simulink model "RotationalPendulum_Nonlinear"  (R2025b)
settings: Solver=VariableStepAuto  StartTime=0.0  StopTime=10  RelTol=1e-3
values from neighbouring files (symbols this model uses):
  eps_v1 = 0.02    [build_sysid_parameters.m]
  eps_v2 = 0.02    [build_sysid_parameters.m]
  p_0 = 0    [build_sysid_parameters.m]
  p_alpha = 33.6175    [build_sysid_parameters.m]
  p_b1 = 744.5341    [build_sysid_parameters.m]
  p_b2 = 0.0670    (= 0.067)    [build_sysid_parameters.m]
  p_c = (l_1 / g) * p_g2    (= 1.14196432212)    [build_sysid_parameters.m]
  p_c1 = 23.9089    [build_sysid_parameters.m]
  p_c2 = 0.2491    [build_sysid_parameters.m]
  p_g1 = 105.6867    [build_sysid_parameters.m]
  p_g2 = 112.0267    [build_sysid_parameters.m]
  p_s_d2 = 0.1836    [build_sysid_parameters.m]
  p_u = 4091.4423    [build_sysid_parameters.m]
  v_s2 = 3.5000    (= 3.5)    [build_sysid_parameters.m]
undefined symbols (not defined in the file or in its folder): theta_1_0_mask, theta_1_dot_0_mask, theta_2_0_mask, theta_2_dot_0_mask
settings Model: Creator=djangovanderplas  LastModifiedBy=thoma
settings DataIOCC: ExternalInput=inputData

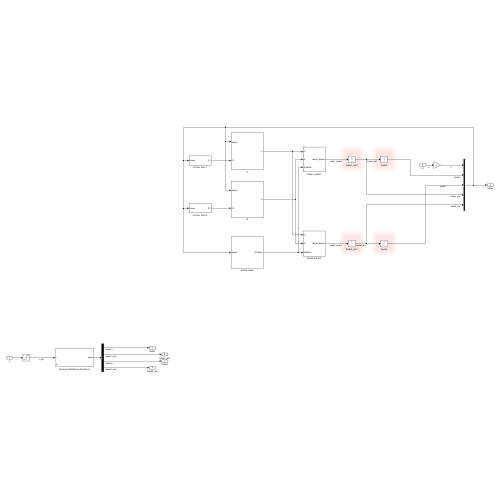
[thumbnail: Simulink's stored preview of the top-level diagram]
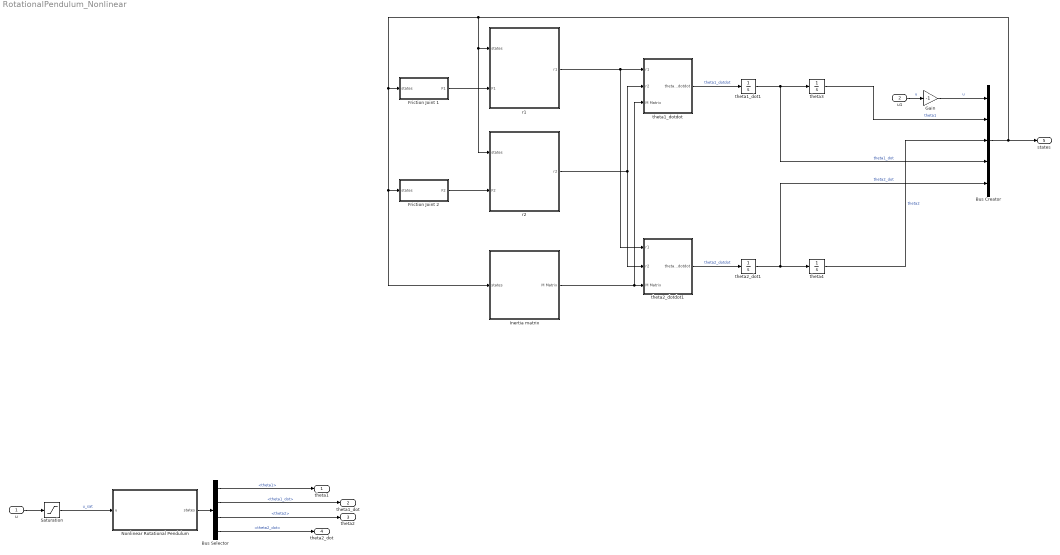
== system RotationalPendulum_Nonlinear ==
  u : Inport
  u1 : Inport  Port=2
  Bus Creator : BusCreator  Inputs=5
  Bus Selector : BusSelector  OutputSignals=theta1,theta1_dot,theta2,theta2_dot
  Friction Joint 1 : Subsystem
  Friction Joint 2 : Subsystem
  Gain : Gain  Gain=-1
  Inertia matrix : Subsystem
  Nonlinear Rotational Pendulum : Subsystem  mask{theta_1_0_mask=pi+0.1, theta_2_0_mask=0, theta_1_dot_0_mask=0, theta_2_dot_0_mask=0}
      mask prompts: theta_1_0_mask "Initial \theta_1 [rad]"; theta_2_0_mask "Initial \theta_2 [rad]"; theta_1_dot_0_mask "Initial \dot\theta_1 [rad]"; theta_2_dot_0_mask "Initial \dot\theta_1 [rad]"
  Saturation : Saturate  UpperLimit=1  LowerLimit=-1
  r1 : Subsystem
  r2 : Subsystem
  theta1_dot1 : Integrator  InitialCondition=theta_1_dot_0_mask
  theta1_dotdot : Subsystem
  theta2_dot1 : Integrator  InitialCondition=theta_2_dot_0_mask
  theta2_dotdot1 : Subsystem
  theta3 : Integrator  InitialCondition=theta_1_0_mask
  theta4 : Integrator  InitialCondition=theta_2_0_mask
  theta1 : Outport
  theta1_dot : Outport  Port=2
  theta2 : Outport  Port=3
  theta2_dot : Outport  Port=4
  states : Outport  Port=5
  wires:
  u/1 -> Saturation/1
  Nonlinear Rotational Pendulum/1(states) -> Bus Selector/1
  Bus Selector/1 -> theta1/1  "<theta1>"
  Bus Selector/3 -> theta2/1  "<theta2>"
  Bus Selector/2 -> theta1_dot/1  "<theta1_dot>"
  Bus Selector/4 -> theta2_dot/1  "<theta2_dot>"
  Saturation/1 -> Nonlinear Rotational Pendulum/1(u)  "u_sat"
  Inertia matrix/1(M Matrix) -> theta2_dotdot1/3(M Matrix), theta1_dotdot/3(M Matrix)
  u1/1 -> Gain/1  "u"
  Friction Joint 1/1(F1) -> r1/2(F1)
  Bus Creator/1 -> Friction Joint 2/1(states), Inertia matrix/1(states), Friction Joint 1/1(states), r1/1(states), r2/1(states), states/1
  theta3/1 -> Bus Creator/2  "theta1"
  theta2_dot1/1 -> theta4/1, Bus Creator/5  "theta2_dot"
  theta1_dotdot/1(theta1_dotdot) -> theta1_dot1/1  "theta1_dotdot"
  Gain/1 -> Bus Creator/1  "u"
  r1/1(r1) -> theta2_dotdot1/1(r1), theta1_dotdot/1(r1)
  theta4/1 -> Bus Creator/3  "theta2"
  r2/1(r2) -> theta2_dotdot1/2(r2), theta1_dotdot/2(r2)
  theta1_dot1/1 -> Bus Creator/4, theta3/1  "theta1_dot"
  Friction Joint 2/1(F2) -> r2/2(F2)
  theta2_dotdot1/1(theta2_dotdot) -> theta2_dot1/1  "theta2_dotdot"

== system RotationalPendulum_Nonlinear/Friction Joint 1 ==
  states : Inport
  Add : Sum
  Bus Selector : BusSelector  OutputSignals=theta1_dot
  Gain : Gain  Gain=p_b1
  Gain1 : Gain  Gain=1/eps_v1
  Gain2 : Gain  Gain=p_c1
  Tanh : Trigonometry  Operator=tanh
  F1 : Outport
  wires:
  states/1 -> Bus Selector/1
  Gain1/1 -> Tanh/1
  Tanh/1 -> Gain2/1
  Add/1 -> F1/1
  Gain2/1 -> Add/1
  Gain/1 -> Add/2
  Bus Selector/1 -> Gain1/1, Gain/1  "<theta1_dot>"

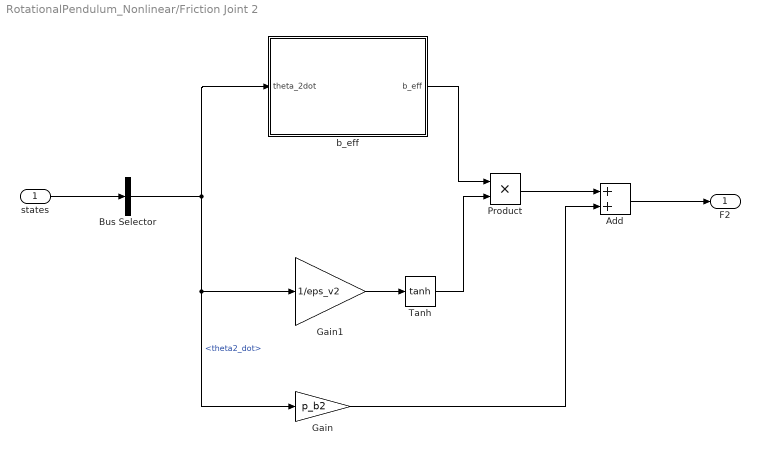
== system RotationalPendulum_Nonlinear/Friction Joint 2 ==
  states : Inport
  Add : Sum
  Bus Selector : BusSelector  OutputSignals=theta2_dot
  Gain : Gain  Gain=p_b2
  Gain1 : Gain  Gain=1/eps_v2
  Product : Product
  Tanh : Trigonometry  Operator=tanh
  b_eff : Subsystem
  F2 : Outport
  wires:
  Bus Selector/1 -> b_eff/1(theta_2dot), Gain/1, Gain1/1  "<theta2_dot>"
  Gain1/1 -> Tanh/1
  Tanh/1 -> Product/2
  Add/1 -> F2/1
  states/1 -> Bus Selector/1
  b_eff/1(b_eff) -> Product/1
  Product/1 -> Add/1
  Gain/1 -> Add/2

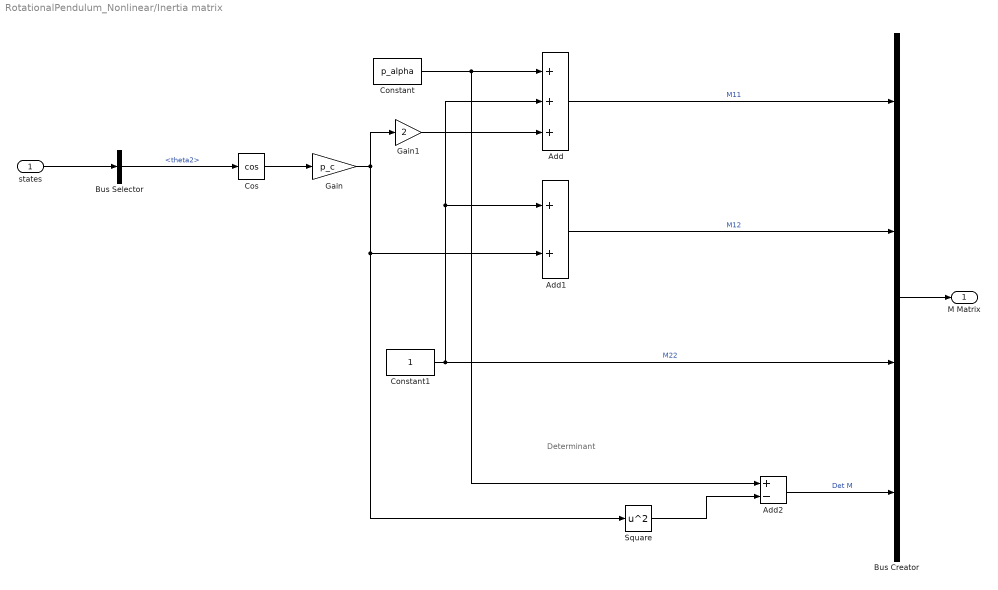
== system RotationalPendulum_Nonlinear/Inertia matrix ==
  note: Determinant
  states : Inport
  Add : Sum  Inputs=+++
  Add1 : Sum
  Add2 : Sum  Inputs=+-
  Bus Creator : BusCreator  Inputs=4
  Bus Selector : BusSelector  OutputSignals=theta2
  Constant : Constant  Value=p_alpha
  Constant1 : Constant
  Cos : Trigonometry  Operator=cos
  Gain : Gain  Gain=p_c
  Gain1 : Gain  Gain=2
  Square : Math  Operator=square
  M Matrix : Outport
  wires:
  states/1 -> Bus Selector/1
  Cos/1 -> Gain/1
  Gain/1 -> Square/1, Add1/2, Gain1/1
  Add/1 -> Bus Creator/1  "M11"
  Constant/1 -> Add2/1, Add/1
  Constant1/1 -> Add/2, Add1/1, Bus Creator/3  "M22"
  Gain1/1 -> Add/3
  Add1/1 -> Bus Creator/2  "M12"
  Add2/1 -> Bus Creator/4  "Det M"
  Bus Selector/1 -> Cos/1  "<theta2>"
  Bus Creator/1 -> M Matrix/1
  Square/1 -> Add2/2

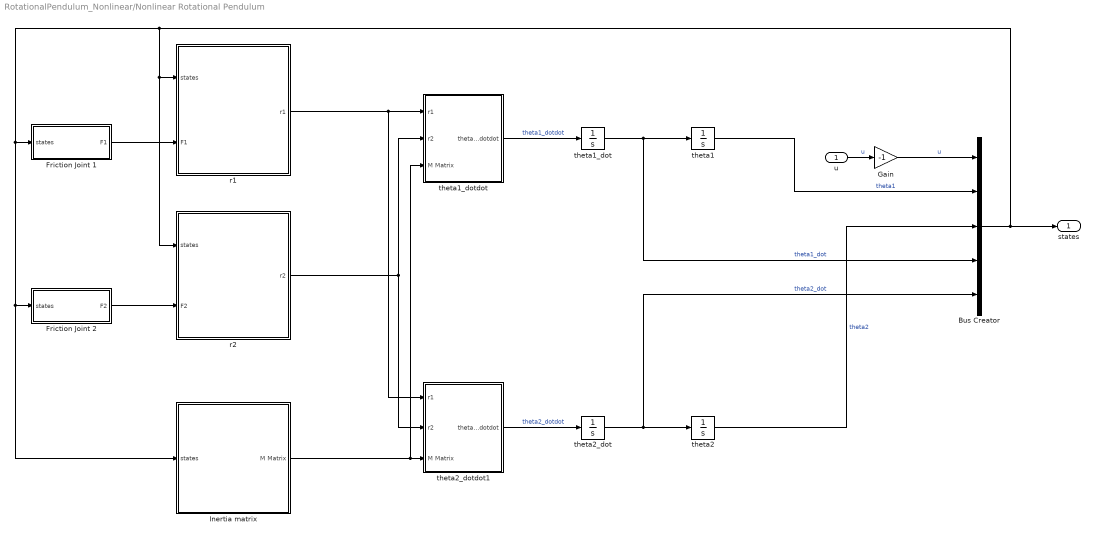
== system RotationalPendulum_Nonlinear/Nonlinear Rotational Pendulum ==
  u : Inport
  Bus Creator : BusCreator  Inputs=5
  Friction Joint 1 : Subsystem
  Friction Joint 2 : Subsystem
  Gain : Gain  Gain=-1
  Inertia matrix : Subsystem
  r1 : Subsystem
  r2 : Subsystem
  theta1 : Integrator  InitialCondition=theta_1_0_mask
  theta1_dot : Integrator  InitialCondition=theta_1_dot_0_mask
  theta1_dotdot : Subsystem
  theta2 : Integrator  InitialCondition=theta_2_0_mask
  theta2_dot : Integrator  InitialCondition=theta_2_dot_0_mask
  theta2_dotdot1 : Subsystem
  states : Outport
  wires:
  Friction Joint 1/1(F1) -> r1/2(F1)
  Friction Joint 2/1(F2) -> r2/2(F2)
  Bus Creator/1 -> Friction Joint 2/1(states), Inertia matrix/1(states), Friction Joint 1/1(states), r1/1(states), r2/1(states), states/1
  u/1 -> Gain/1  "u"
  theta1/1 -> Bus Creator/2  "theta1"
  theta2/1 -> Bus Creator/3  "theta2"
  theta2_dot/1 -> theta2/1, Bus Creator/5  "theta2_dot"
  r1/1(r1) -> theta2_dotdot1/1(r1), theta1_dotdot/1(r1)
  r2/1(r2) -> theta2_dotdot1/2(r2), theta1_dotdot/2(r2)
  Inertia matrix/1(M Matrix) -> theta2_dotdot1/3(M Matrix), theta1_dotdot/3(M Matrix)
  theta1_dotdot/1(theta1_dotdot) -> theta1_dot/1  "theta1_dotdot"
  theta1_dot/1 -> Bus Creator/4, theta1/1  "theta1_dot"
  theta2_dotdot1/1(theta2_dotdot) -> theta2_dot/1  "theta2_dotdot"
  Gain/1 -> Bus Creator/1  "u"

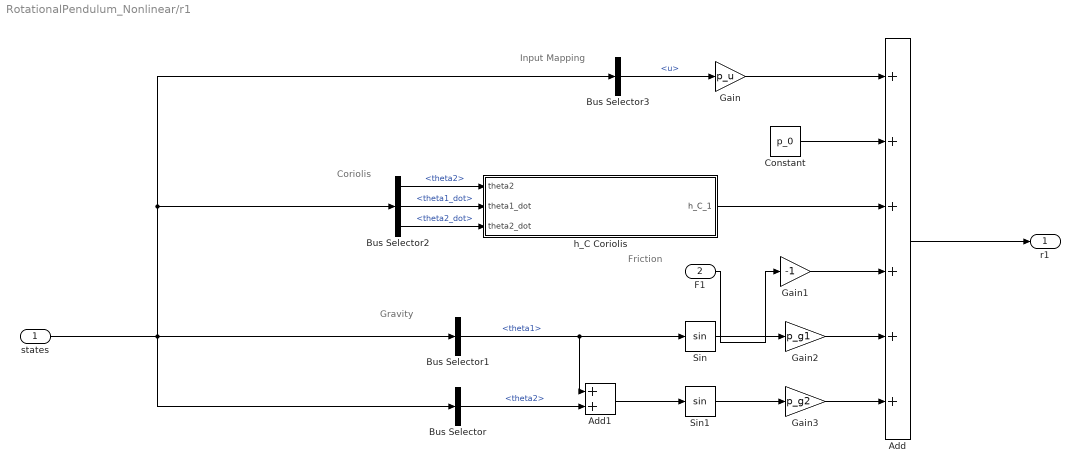
== system RotationalPendulum_Nonlinear/r1 ==
  note: Coriolis
  note: Input Mapping
  note: Friction
  note: Gravity
  states : Inport
  F1 : Inport  Port=2
  Add : Sum  Inputs=++++++
  Add1 : Sum
  Bus Selector : BusSelector  OutputSignals=theta2
  Bus Selector1 : BusSelector  OutputSignals=theta1
  Bus Selector2 : BusSelector  OutputSignals=theta2,theta1_dot,theta2_dot
  Bus Selector3 : BusSelector  OutputSignals=u
  Constant : Constant  Value=p_0
  Gain : Gain  Gain=p_u
  Gain1 : Gain  Gain=-1
  Gain2 : Gain  Gain=p_g1
  Gain3 : Gain  Gain=p_g2
  Sin : Trigonometry
  Sin1 : Trigonometry
  h_C Coriolis : Subsystem
  r1 : Outport
  wires:
  Add/1 -> r1/1
  Bus Selector3/1 -> Gain/1  "<u>"
  Gain/1 -> Add/1
  Constant/1 -> Add/2
  Bus Selector1/1 -> Add1/1, Sin/1  "<theta1>"
  h_C Coriolis/1(h_C_1) -> Add/3
  Gain1/1 -> Add/4
  F1/1 -> Gain1/1
  Sin/1 -> Gain2/1
  Gain2/1 -> Add/5
  Bus Selector/1 -> Add1/2  "<theta2>"
  Add1/1 -> Sin1/1
  Sin1/1 -> Gain3/1
  Gain3/1 -> Add/6
  states/1 -> Bus Selector3/1, Bus Selector2/1, Bus Selector1/1, Bus Selector/1
  Bus Selector2/2 -> h_C Coriolis/2(theta1_dot)  "<theta1_dot>"
  Bus Selector2/3 -> h_C Coriolis/3(theta2_dot)  "<theta2_dot>"
  Bus Selector2/1 -> h_C Coriolis/1(theta2)  "<theta2>"

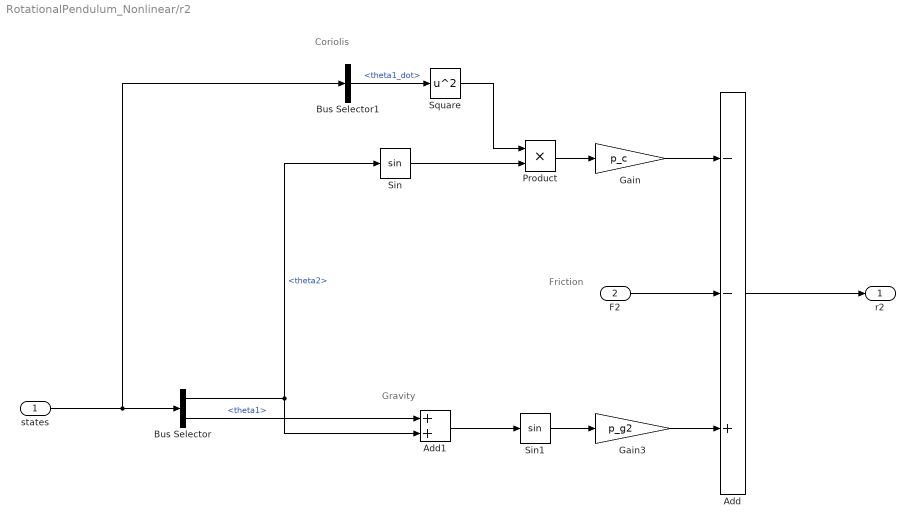
== system RotationalPendulum_Nonlinear/r2 ==
  note: Gravity
  note: Coriolis
  note: Friction
  states : Inport
  F2 : Inport  Port=2
  Add : Sum  Inputs=--+
  Add1 : Sum
  Bus Selector : BusSelector  OutputSignals=theta2,theta1
  Bus Selector1 : BusSelector  OutputSignals=theta1_dot
  Gain : Gain  Gain=p_c
  Gain3 : Gain  Gain=p_g2
  Product : Product
  Sin : Trigonometry
  Sin1 : Trigonometry
  Square : Math  Operator=square
  r2 : Outport
  wires:
  Add/1 -> r2/1
  F2/1 -> Add/2
  Add1/1 -> Sin1/1
  Sin1/1 -> Gain3/1
  Gain3/1 -> Add/3
  Gain/1 -> Add/1
  Product/1 -> Gain/1
  Square/1 -> Product/1
  Sin/1 -> Product/2
  states/1 -> Bus Selector1/1, Bus Selector/1
  Bus Selector/1 -> Add1/2, Sin/1  "<theta2>"
  Bus Selector/2 -> Add1/1  "<theta1>"
  Bus Selector1/1 -> Square/1  "<theta1_dot>"

== system RotationalPendulum_Nonlinear/theta1_dotdot ==
  r1 : Inport
  r2 : Inport  Port=2
  M Matrix : Inport  Port=3
  Bus Selector : BusSelector  OutputSignals=M12,Det M
  Divide : Product  Inputs=*/
  Product : Product
  Subtract : Sum  Inputs=+-
  theta1_dotdot : Outport
  wires:
  r1/1 -> Subtract/1
  Product/1 -> Subtract/2
  r2/1 -> Product/2
  M Matrix/1 -> Bus Selector/1
  Bus Selector/1 -> Product/1  "<M12>"
  Subtract/1 -> Divide/1
  Bus Selector/2 -> Divide/2  "<Det M>"
  Divide/1 -> theta1_dotdot/1

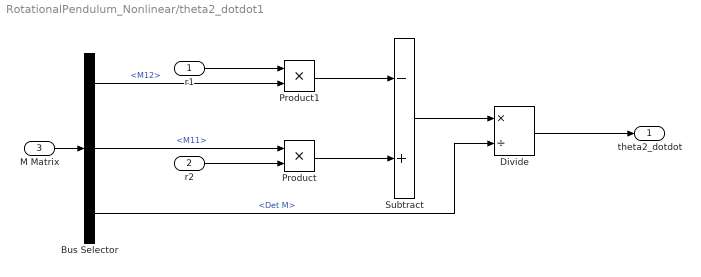
== system RotationalPendulum_Nonlinear/theta2_dotdot1 ==
  r1 : Inport
  r2 : Inport  Port=2
  M Matrix : Inport  Port=3
  Bus Selector : BusSelector  OutputSignals=M12,M11,Det M
  Divide : Product  Inputs=*/
  Product : Product
  Product1 : Product
  Subtract : Sum  Inputs=-+
  theta2_dotdot : Outport
  wires:
  M Matrix/1 -> Bus Selector/1
  Divide/1 -> theta2_dotdot/1
  Bus Selector/3 -> Divide/2  "<Det M>"
  Subtract/1 -> Divide/1
  r2/1 -> Product/2
  Product/1 -> Subtract/2
  Product1/1 -> Subtract/1
  r1/1 -> Product1/1
  Bus Selector/1 -> Product1/2  "<M12>"
  Bus Selector/2 -> Product/1  "<M11>"

== system RotationalPendulum_Nonlinear/Friction Joint 2/b_eff ==
  theta_2dot : Inport
  Add : Sum
  Constant : Constant  Value=p_c2
  Exp : Math
  Gain : Gain  Gain=-1
  Gain1 : Gain  Gain=(1/v_s2)
  Gain2 : Gain  Gain=p_s_d2
  Square : Math  Operator=square
  b_eff : Outport
  wires:
  Add/1 -> b_eff/1
  Gain1/1 -> Square/1
  Constant/1 -> Add/2
  Exp/1 -> Gain2/1
  theta_2dot/1 -> Gain1/1
  Gain2/1 -> Add/1
  Square/1 -> Gain/1
  Gain/1 -> Exp/1

== system RotationalPendulum_Nonlinear/Nonlinear Rotational Pendulum/Friction Joint 1 ==
  states : Inport
  Add : Sum
  Bus Selector : BusSelector  OutputSignals=theta1_dot
  Gain : Gain  Gain=p_b1
  Gain1 : Gain  Gain=1/eps_v1
  Gain2 : Gain  Gain=p_c1
  Tanh : Trigonometry  Operator=tanh
  F1 : Outport
  wires:
  states/1 -> Bus Selector/1
  Gain1/1 -> Tanh/1
  Tanh/1 -> Gain2/1
  Add/1 -> F1/1
  Gain2/1 -> Add/1
  Gain/1 -> Add/2
  Bus Selector/1 -> Gain1/1, Gain/1  "<theta1_dot>"

== system RotationalPendulum_Nonlinear/Nonlinear Rotational Pendulum/Friction Joint 2 ==
  states : Inport
  Add : Sum
  Bus Selector : BusSelector  OutputSignals=theta2_dot
  Gain : Gain  Gain=p_b2
  Gain1 : Gain  Gain=1/eps_v2
  Product : Product
  Tanh : Trigonometry  Operator=tanh
  b_eff : Subsystem
  F2 : Outport
  wires:
  Bus Selector/1 -> b_eff/1(theta_2dot), Gain/1, Gain1/1  "<theta2_dot>"
  Gain1/1 -> Tanh/1
  Tanh/1 -> Product/2
  Add/1 -> F2/1
  states/1 -> Bus Selector/1
  b_eff/1(b_eff) -> Product/1
  Product/1 -> Add/1
  Gain/1 -> Add/2

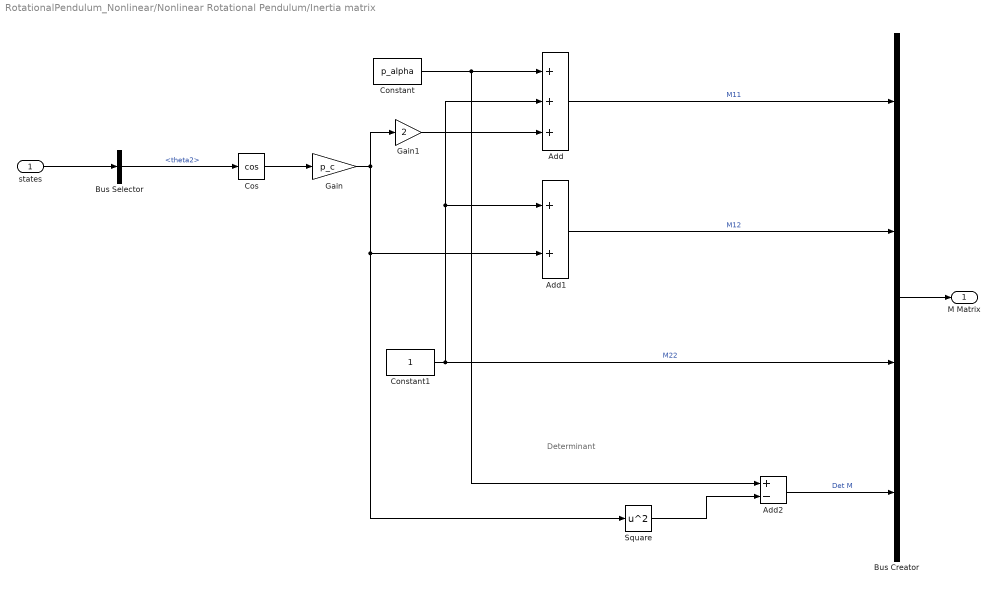
== system RotationalPendulum_Nonlinear/Nonlinear Rotational Pendulum/Inertia matrix ==
  note: Determinant
  states : Inport
  Add : Sum  Inputs=+++
  Add1 : Sum
  Add2 : Sum  Inputs=+-
  Bus Creator : BusCreator  Inputs=4
  Bus Selector : BusSelector  OutputSignals=theta2
  Constant : Constant  Value=p_alpha
  Constant1 : Constant
  Cos : Trigonometry  Operator=cos
  Gain : Gain  Gain=p_c
  Gain1 : Gain  Gain=2
  Square : Math  Operator=square
  M Matrix : Outport
  wires:
  states/1 -> Bus Selector/1
  Cos/1 -> Gain/1
  Gain/1 -> Square/1, Add1/2, Gain1/1
  Add/1 -> Bus Creator/1  "M11"
  Constant/1 -> Add2/1, Add/1
  Constant1/1 -> Add/2, Add1/1, Bus Creator/3  "M22"
  Gain1/1 -> Add/3
  Add1/1 -> Bus Creator/2  "M12"
  Add2/1 -> Bus Creator/4  "Det M"
  Bus Selector/1 -> Cos/1  "<theta2>"
  Bus Creator/1 -> M Matrix/1
  Square/1 -> Add2/2

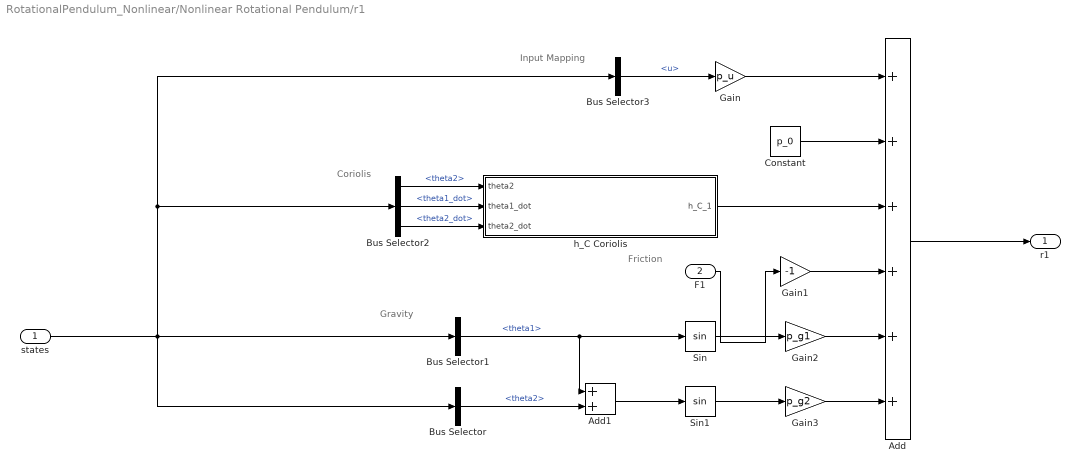
== system RotationalPendulum_Nonlinear/Nonlinear Rotational Pendulum/r1 ==
  note: Coriolis
  note: Input Mapping
  note: Friction
  note: Gravity
  states : Inport
  F1 : Inport  Port=2
  Add : Sum  Inputs=++++++
  Add1 : Sum
  Bus Selector : BusSelector  OutputSignals=theta2
  Bus Selector1 : BusSelector  OutputSignals=theta1
  Bus Selector2 : BusSelector  OutputSignals=theta2,theta1_dot,theta2_dot
  Bus Selector3 : BusSelector  OutputSignals=u
  Constant : Constant  Value=p_0
  Gain : Gain  Gain=p_u
  Gain1 : Gain  Gain=-1
  Gain2 : Gain  Gain=p_g1
  Gain3 : Gain  Gain=p_g2
  Sin : Trigonometry
  Sin1 : Trigonometry
  h_C Coriolis : Subsystem
  r1 : Outport
  wires:
  Add/1 -> r1/1
  Bus Selector3/1 -> Gain/1  "<u>"
  Gain/1 -> Add/1
  Constant/1 -> Add/2
  Bus Selector1/1 -> Add1/1, Sin/1  "<theta1>"
  h_C Coriolis/1(h_C_1) -> Add/3
  Gain1/1 -> Add/4
  F1/1 -> Gain1/1
  Sin/1 -> Gain2/1
  Gain2/1 -> Add/5
  Bus Selector/1 -> Add1/2  "<theta2>"
  Add1/1 -> Sin1/1
  Sin1/1 -> Gain3/1
  Gain3/1 -> Add/6
  states/1 -> Bus Selector3/1, Bus Selector2/1, Bus Selector1/1, Bus Selector/1
  Bus Selector2/2 -> h_C Coriolis/2(theta1_dot)  "<theta1_dot>"
  Bus Selector2/3 -> h_C Coriolis/3(theta2_dot)  "<theta2_dot>"
  Bus Selector2/1 -> h_C Coriolis/1(theta2)  "<theta2>"

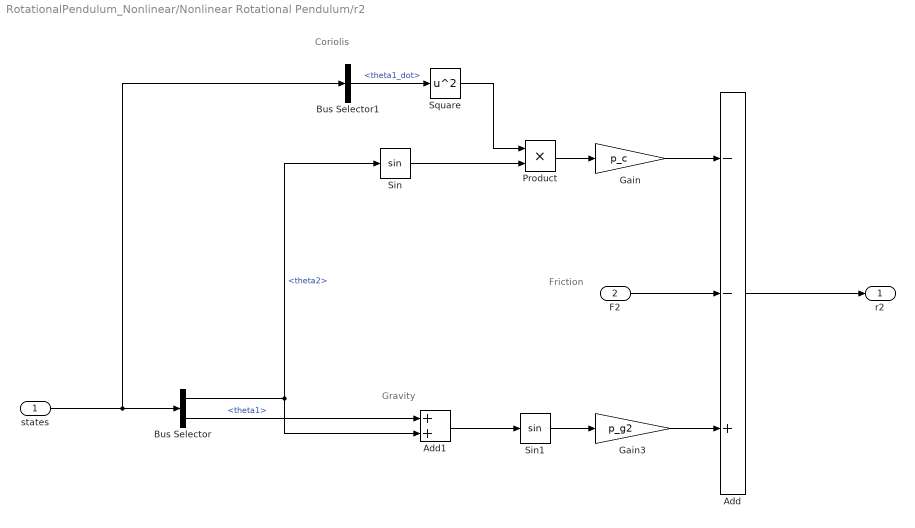
== system RotationalPendulum_Nonlinear/Nonlinear Rotational Pendulum/r2 ==
  note: Gravity
  note: Coriolis
  note: Friction
  states : Inport
  F2 : Inport  Port=2
  Add : Sum  Inputs=--+
  Add1 : Sum
  Bus Selector : BusSelector  OutputSignals=theta2,theta1
  Bus Selector1 : BusSelector  OutputSignals=theta1_dot
  Gain : Gain  Gain=p_c
  Gain3 : Gain  Gain=p_g2
  Product : Product
  Sin : Trigonometry
  Sin1 : Trigonometry
  Square : Math  Operator=square
  r2 : Outport
  wires:
  Add/1 -> r2/1
  F2/1 -> Add/2
  Add1/1 -> Sin1/1
  Sin1/1 -> Gain3/1
  Gain3/1 -> Add/3
  Gain/1 -> Add/1
  Product/1 -> Gain/1
  Square/1 -> Product/1
  Sin/1 -> Product/2
  states/1 -> Bus Selector1/1, Bus Selector/1
  Bus Selector/1 -> Add1/2, Sin/1  "<theta2>"
  Bus Selector/2 -> Add1/1  "<theta1>"
  Bus Selector1/1 -> Square/1  "<theta1_dot>"

== system RotationalPendulum_Nonlinear/Nonlinear Rotational Pendulum/theta1_dotdot ==
  r1 : Inport
  r2 : Inport  Port=2
  M Matrix : Inport  Port=3
  Bus Selector : BusSelector  OutputSignals=M12,Det M
  Divide : Product  Inputs=*/
  Product : Product
  Subtract : Sum  Inputs=+-
  theta1_dotdot : Outport
  wires:
  r1/1 -> Subtract/1
  Product/1 -> Subtract/2
  r2/1 -> Product/2
  M Matrix/1 -> Bus Selector/1
  Bus Selector/1 -> Product/1  "<M12>"
  Subtract/1 -> Divide/1
  Bus Selector/2 -> Divide/2  "<Det M>"
  Divide/1 -> theta1_dotdot/1

== system RotationalPendulum_Nonlinear/Nonlinear Rotational Pendulum/theta2_dotdot1 ==
  r1 : Inport
  r2 : Inport  Port=2
  M Matrix : Inport  Port=3
  Bus Selector : BusSelector  OutputSignals=M12,M11,Det M
  Divide : Product  Inputs=*/
  Product : Product
  Product1 : Product
  Subtract : Sum  Inputs=-+
  theta2_dotdot : Outport
  wires:
  M Matrix/1 -> Bus Selector/1
  Divide/1 -> theta2_dotdot/1
  Bus Selector/3 -> Divide/2  "<Det M>"
  Subtract/1 -> Divide/1
  r2/1 -> Product/2
  Product/1 -> Subtract/2
  Product1/1 -> Subtract/1
  r1/1 -> Product1/1
  Bus Selector/1 -> Product1/2  "<M12>"
  Bus Selector/2 -> Product/1  "<M11>"

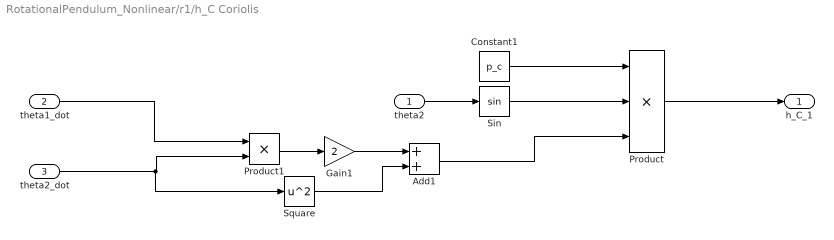
== system RotationalPendulum_Nonlinear/r1/h_C Coriolis ==
  theta2 : Inport
  theta1_dot : Inport  Port=2
  theta2_dot : Inport  Port=3
  Add1 : Sum
  Constant1 : Constant  Value=p_c
  Gain1 : Gain  Gain=2
  Product : Product  Inputs=3
  Product1 : Product
  Sin : Trigonometry
  Square : Math  Operator=square
  h_C_1 : Outport
  wires:
  Gain1/1 -> Add1/1
  theta2/1 -> Sin/1
  Constant1/1 -> Product/1
  Product1/1 -> Gain1/1
  Product/1 -> h_C_1/1
  theta2_dot/1 -> Square/1, Product1/2
  Add1/1 -> Product/3
  theta1_dot/1 -> Product1/1
  Square/1 -> Add1/2
  Sin/1 -> Product/2

== system RotationalPendulum_Nonlinear/Nonlinear Rotational Pendulum/Friction Joint 2/b_eff ==
  theta_2dot : Inport
  Add : Sum
  Constant : Constant  Value=p_c2
  Exp : Math
  Gain : Gain  Gain=-1
  Gain1 : Gain  Gain=(1/v_s2)
  Gain2 : Gain  Gain=p_s_d2
  Square : Math  Operator=square
  b_eff : Outport
  wires:
  Add/1 -> b_eff/1
  Gain1/1 -> Square/1
  Constant/1 -> Add/2
  Exp/1 -> Gain2/1
  theta_2dot/1 -> Gain1/1
  Gain2/1 -> Add/1
  Square/1 -> Gain/1
  Gain/1 -> Exp/1

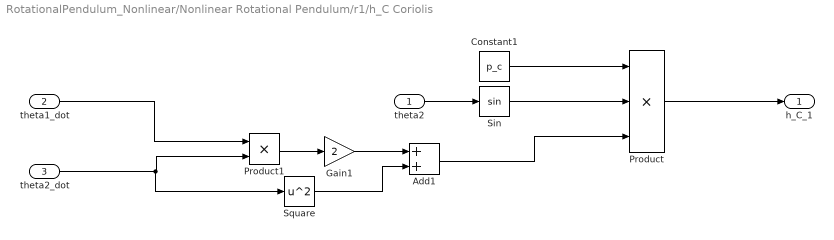
== system RotationalPendulum_Nonlinear/Nonlinear Rotational Pendulum/r1/h_C Coriolis ==
  theta2 : Inport
  theta1_dot : Inport  Port=2
  theta2_dot : Inport  Port=3
  Add1 : Sum
  Constant1 : Constant  Value=p_c
  Gain1 : Gain  Gain=2
  Product : Product  Inputs=3
  Product1 : Product
  Sin : Trigonometry
  Square : Math  Operator=square
  h_C_1 : Outport
  wires:
  Gain1/1 -> Add1/1
  theta2/1 -> Sin/1
  Constant1/1 -> Product/1
  Product1/1 -> Gain1/1
  Product/1 -> h_C_1/1
  theta2_dot/1 -> Square/1, Product1/2
  Add1/1 -> Product/3
  theta1_dot/1 -> Product1/1
  Square/1 -> Add1/2
  Sin/1 -> Product/2
